simulink model "AuE881_HW5_Zhai_Kexuan_BicycleModel"  (R2019a)
settings: Solver=ode15s  StartTime=0.0  StopTime=15  RelTol=1e-3
values from neighbouring files (symbols this model uses):
  a = wb-b    (= 1.4375)    [AuE881_HW5_Zhai_Kexuan_HW5_initialization.m]
  Af = 2.34    [AuE881_HW5_Zhai_Kexuan_HW5_initialization.m]
  b = wb*0.5    (= 1.4375)    [AuE881_HW5_Zhai_Kexuan_HW5_initialization.m]
  Cd = 0.23    [AuE881_HW5_Zhai_Kexuan_HW5_initialization.m]
  Crr = 0.009    [AuE881_HW5_Zhai_Kexuan_HW5_initialization.m]
  delta = 15*pi/180    (= 0.261799387799)    [AuE881_HW5_Zhai_Kexuan_HW5_initialization.m]
  Fz1 = Fz*b/wb    (= 8829)    [AuE881_HW5_Zhai_Kexuan_HW5_initialization.m]
  Fz2 = Fz - Fz1    (= 8829)    [AuE881_HW5_Zhai_Kexuan_HW5_initialization.m]
  g = 9.81    [AuE881_HW5_Zhai_Kexuan_HW5_initialization.m]
  iniPsiDot = 0    [AuE881_HW5_Zhai_Kexuan_HW5_initialization.m]
  iniU = 10    [AuE881_HW5_Zhai_Kexuan_HW5_initialization.m]
  iniV = -10    [AuE881_HW5_Zhai_Kexuan_HW5_initialization.m]
  Jz = 0.9*m*(length/2)^2    (= 8923.62258)    [AuE881_HW5_Zhai_Kexuan_HW5_initialization.m]
  m = 1800    [AuE881_HW5_Zhai_Kexuan_HW5_initialization.m]
  rho_air = 1.26    [AuE881_HW5_Zhai_Kexuan_HW5_initialization.m]
  tireVelDesired = 20    [AuE881_HW5_Zhai_Kexuan_HW5_initialization.m]
settings Model: Creator=paredis  LastModifiedBy=kzhai

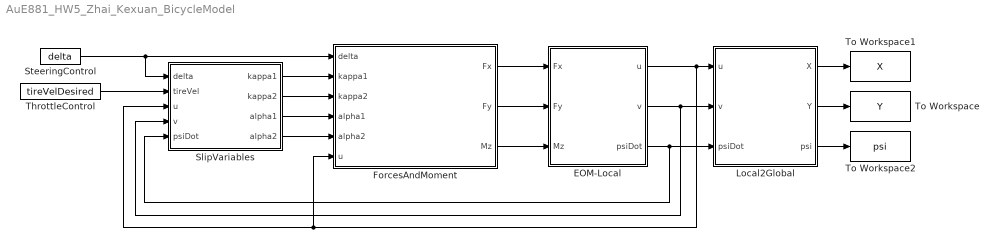
== system AuE881_HW5_Zhai_Kexuan_BicycleModel ==
  EOM-Local : Subsystem
  ForcesAndMoment : Subsystem
  Local2Global : Subsystem
  SlipVariables : Subsystem
  SteeringControl : Constant  Value=delta
  ThrottleControl : Constant  Value=tireVelDesired
  To Workspace : ToWorkspace  VariableName=Y  SaveFormat=Timeseries  SampleTime=-1
  To Workspace1 : ToWorkspace  VariableName=X  SaveFormat=Timeseries  SampleTime=-1
  To Workspace2 : ToWorkspace  VariableName=psi  SaveFormat=Timeseries  SampleTime=-1
  wires:
  EOM-Local/3(psiDot) -> SlipVariables/5(psiDot), Local2Global/3(psiDot)
  EOM-Local/2(v) -> SlipVariables/4(v), Local2Global/2(v)
  Local2Global/2(Y) -> To Workspace/1
  Local2Global/1(X) -> To Workspace1/1
  Local2Global/3(psi) -> To Workspace2/1
  SteeringControl/1 -> ForcesAndMoment/1(delta), SlipVariables/1(delta)
  SlipVariables/3(alpha1) -> ForcesAndMoment/4(alpha1)
  SlipVariables/4(alpha2) -> ForcesAndMoment/5(alpha2)
  ForcesAndMoment/1(Fx) -> EOM-Local/1(Fx)
  ForcesAndMoment/2(Fy) -> EOM-Local/2(Fy)
  ForcesAndMoment/3(Mz) -> EOM-Local/3(Mz)
  SlipVariables/2(kappa2) -> ForcesAndMoment/3(kappa2)
  SlipVariables/1(kappa1) -> ForcesAndMoment/2(kappa1)
  ThrottleControl/1 -> SlipVariables/2(tireVel)
  EOM-Local/1(u) -> Local2Global/1(u), ForcesAndMoment/6(u), SlipVariables/3(u)

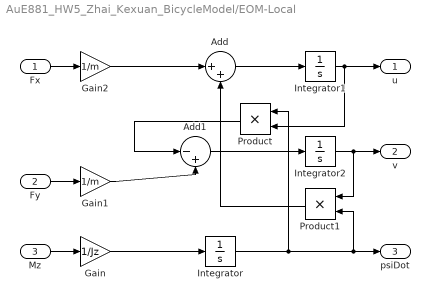
== system AuE881_HW5_Zhai_Kexuan_BicycleModel/EOM-Local ==
  Fx : Inport
  Fy : Inport  Port=2
  Mz : Inport  Port=3
  Add : Sum  Inputs=|++
  Add1 : Sum  Inputs=|-+
  Gain : Gain  Gain=1/Jz
  Gain1 : Gain  Gain=1/m
  Gain2 : Gain  Gain=1/m
  Integrator : Integrator  InitialCondition=iniPsiDot
  Integrator1 : Integrator  InitialCondition=iniU
  Integrator2 : Integrator  InitialCondition=iniV
  Product : Product
  Product1 : Product
  u : Outport
  v : Outport  Port=2
  psiDot : Outport  Port=3
  wires:
  Integrator1/1 -> u/1, Product/2
  Integrator2/1 -> Product1/1, v/1
  Product/1 -> Add1/1
  Gain1/1 -> Add1/2
  Product1/1 -> Add/2
  Gain/1 -> Integrator/1
  Add/1 -> Integrator1/1
  Mz/1 -> Gain/1
  Gain2/1 -> Add/1
  Fy/1 -> Gain1/1
  Integrator/1 -> psiDot/1, Product1/2, Product/1
  Fx/1 -> Gain2/1
  Add1/1 -> Integrator2/1

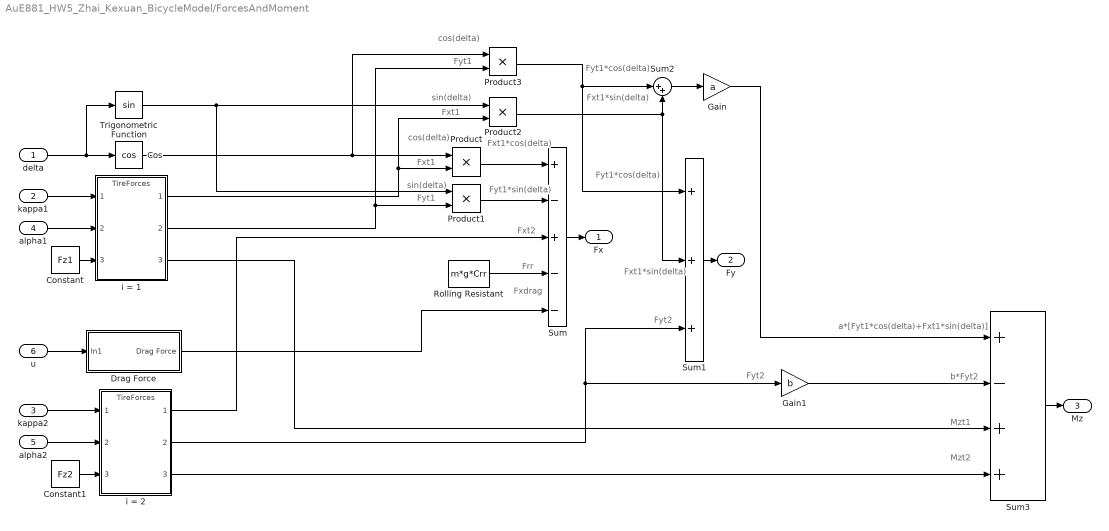
== system AuE881_HW5_Zhai_Kexuan_BicycleModel/ForcesAndMoment ==
  note: sin(delta)
  note: cos(delta)
  note: Fxt1
  note: Fxt1
  note: Fxt1*sin(delta)
  note: cos(delta)
  note: Fyt1
  note: sin(delta)
  note: Fyt1
  note: Fyt1*cos(delta)
  note: a*[Fyt1*cos(delta)+Fxt1*sin(delta)]
  note: Fxt2
  note: Frr
  note: Fxdrag
  note: Fyt2
  note: Fyt2
  note: Mzt1
  note: Mzt2
  note: b*Fyt2
  note: Fyt1*cos(delta)
  note: Fxt1*sin(delta)
  note: Fxt1*cos(delta)
  note: Fyt1*sin(delta)
  delta : Inport
  kappa1 : Inport  Port=2
  kappa2 : Inport  Port=3
  alpha1 : Inport  Port=4
  alpha2 : Inport  Port=5
  u : Inport  Port=6
  Constant : Constant  Value=Fz1
  Constant1 : Constant  Value=Fz2
  Cos : Trigonometry  Operator=cos
  Drag Force : Subsystem
  Gain : Gain  Gain=a
  Gain1 : Gain  Gain=b
  Product{,1..3} (4 alike) : Product
  Rolling Resistant : Constant  Value=m*g*Crr
  Sum : Sum  Inputs=+-+--
  Sum1 : Sum  Inputs=+++
  Sum2 : Sum  Inputs=|++
  Sum3 : Sum  Inputs=+-++
  Trigonometric Function : Trigonometry
  i = 1 : ModelReference  ModelNameDialog=TireForces  SimulationMode=Normal  ModelReferenceVersion=1.12
  i = 2 : ModelReference  ModelNameDialog=TireForces  SimulationMode=Normal  ModelReferenceVersion=1.12
  Fx : Outport
  Fy : Outport  Port=2
  Mz : Outport  Port=3
  wires:
  i = 1/3 -> Sum3/3
  Sum3/1 -> Mz/1
  Gain1/1 -> Sum3/2
  Drag Force/1(Drag Force) -> Sum/5
  delta/1 -> Cos/1, Trigonometric Function/1
  i = 2/1 -> Sum/3
  Cos/1 -> Product3/1, Product/1
  Product2/1 -> Sum1/2, Sum2/2
  Sum1/1 -> Fy/1
  Sum2/1 -> Gain/1
  Product1/1 -> Sum/2
  alpha1/1 -> i = 1/2
  Gain/1 -> Sum3/1
  i = 1/2 -> Product1/2, Product3/2
  i = 2/2 -> Gain1/1, Sum1/3
  Product/1 -> Sum/1
  Constant1/1 -> i = 2/3
  Sum/1 -> Fx/1
  Trigonometric Function/1 -> Product2/1, Product1/1
  i = 2/3 -> Sum3/4
  Rolling Resistant/1 -> Sum/4
  Constant/1 -> i = 1/3
  alpha2/1 -> i = 2/2
  kappa2/1 -> i = 2/1
  kappa1/1 -> i = 1/1
  Product3/1 -> Sum2/1, Sum1/1
  i = 1/1 -> Product/2, Product2/2
  u/1 -> Drag Force/1(In1)

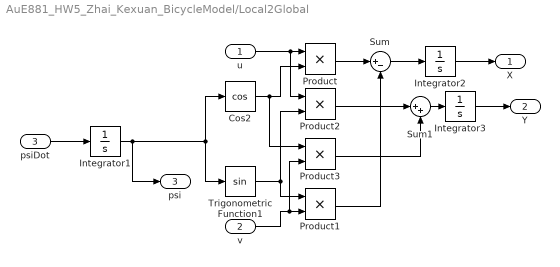
== system AuE881_HW5_Zhai_Kexuan_BicycleModel/Local2Global ==
  u : Inport
  v : Inport  Port=2
  psiDot : Inport  Port=3
  Cos2 : Trigonometry  Operator=cos
  Integrator1 : Integrator
  Integrator2 : Integrator
  Integrator3 : Integrator
  Product{,1..3} (4 alike) : Product
  Sum : Sum  Inputs=|+-
  Sum1 : Sum  Inputs=|++
  Trigonometric Function1 : Trigonometry
  X : Outport
  Y : Outport  Port=2
  psi : Outport  Port=3
  wires:
  psiDot/1 -> Integrator1/1
  u/1 -> Product2/1, Product/1
  Integrator1/1 -> Cos2/1, Trigonometric Function1/1, psi/1
  v/1 -> Product3/2, Product1/2
  Sum1/1 -> Integrator3/1
  Cos2/1 -> Product3/1, Product/2
  Integrator2/1 -> X/1
  Product1/1 -> Sum/2
  Product2/1 -> Sum1/1
  Product/1 -> Sum/1
  Sum/1 -> Integrator2/1
  Trigonometric Function1/1 -> Product1/1, Product2/2
  Product3/1 -> Sum1/2
  Integrator3/1 -> Y/1

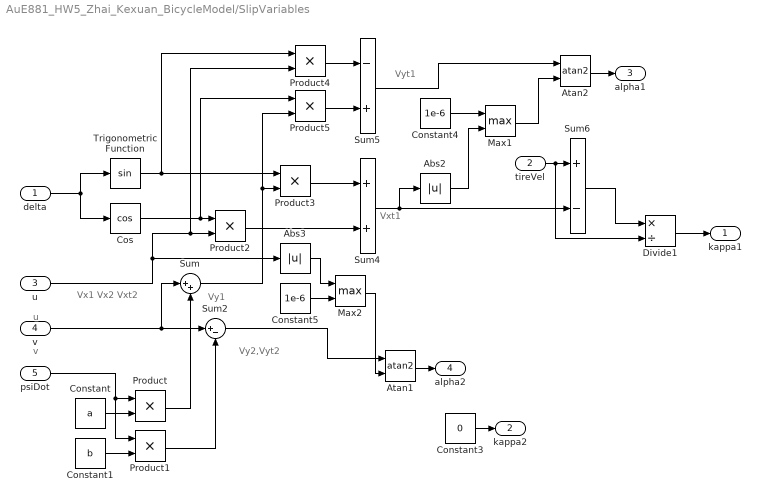
== system AuE881_HW5_Zhai_Kexuan_BicycleModel/SlipVariables ==
  note: Vyt1
  note: Vy2,Vyt2
  note: Vxt1
  note: Vx1 Vx2 Vxt2
  note: Vy1
  note: v
  note: u
  delta : Inport
  tireVel : Inport  Port=2
  u : Inport  Port=3
  v : Inport  Port=4
  psiDot : Inport  Port=5
  Abs2 : Abs
  Abs3 : Abs
  Atan1 : Trigonometry  Operator=atan2
  Atan2 : Trigonometry  Operator=atan2
  Constant : Constant  Value=a
  Constant1 : Constant  Value=b
  Constant3 : Constant  Value=0
  Constant4 : Constant  Value=1e-6
  Constant5 : Constant  Value=1e-6
  Cos : Trigonometry  Operator=cos
  Divide1 : Product  Inputs=*/
  Max1 : MinMax  Function=max  Inputs=2
  Max2 : MinMax  Function=max  Inputs=2
  Product{,1..5} (6 alike) : Product
  Sum : Sum  Inputs=|++
  Sum2 : Sum  Inputs=|+-
  Sum4 : Sum
  Sum5 : Sum  Inputs=-+
  Sum6 : Sum  Inputs=+-
  Trigonometric Function : Trigonometry
  kappa1 : Outport
  kappa2 : Outport  Port=2
  alpha1 : Outport  Port=3
  alpha2 : Outport  Port=4
  wires:
  Sum4/1 -> Abs2/1, Sum6/2
  v/1 -> Sum/1, Sum2/1
  Product1/1 -> Sum2/2
  Sum6/1 -> Divide1/1
  Sum5/1 -> Atan2/1
  Sum/1 -> Product5/2, Product3/2
  Atan1/1 -> alpha2/1
  Atan2/1 -> alpha1/1
  Cos/1 -> Product5/1, Product2/1
  tireVel/1 -> Divide1/2, Sum6/1
  Product5/1 -> Sum5/2
  Product/1 -> Sum/2
  u/1 -> Product4/2, Product2/2, Abs3/1
  Product3/1 -> Sum4/1
  Product2/1 -> Sum4/2
  Trigonometric Function/1 -> Product4/1, Product3/1
  Constant1/1 -> Product1/2
  Sum2/1 -> Atan1/1
  delta/1 -> Cos/1, Trigonometric Function/1
  psiDot/1 -> Product1/1, Product/1
  Constant/1 -> Product/2
  Product4/1 -> Sum5/1
  Divide1/1 -> kappa1/1
  Constant3/1 -> kappa2/1
  Constant4/1 -> Max1/1
  Abs2/1 -> Max1/2
  Max1/1 -> Atan2/2
  Constant5/1 -> Max2/2
  Abs3/1 -> Max2/1
  Max2/1 -> Atan1/2

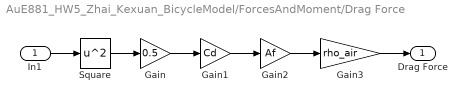
== system AuE881_HW5_Zhai_Kexuan_BicycleModel/ForcesAndMoment/Drag Force ==
  In1 : Inport
  Gain : Gain  Gain=0.5
  Gain1 : Gain  Gain=Cd
  Gain2 : Gain  Gain=Af
  Gain3 : Gain  Gain=rho_air
  Square : Math  Operator=square  SaturateOnIntegerOverflow=on
  Drag Force : Outport
  wires:
  Gain/1 -> Gain1/1
  Gain1/1 -> Gain2/1
  Gain2/1 -> Gain3/1
  In1/1 -> Square/1
  Square/1 -> Gain/1
  Gain3/1 -> Drag Force/1
